simulink model "euler2"  (R2025a)
settings: Solver=VariableStepAuto  StartTime=0.0  StopTime=10.0  RelTol=1e-3
values from neighbouring files (symbols this model uses):
  h = 0.1    [ejemplo_NOlineal_RK4.m]    (also in euler_explicita.m = (tf - t0)/n; euler_explicito.m = (tf - t0)/n; euler_midpoint.m = (tf - t0)/n; examplecrk4.m)
  y0 = 1    [ExampleEuler.m]    (also in ejemplo_NOlineal_RK4.m; examplecrk4.m; exmapleEuler2.m; lineal_RK4.m)
settings Model: Creator=a.diteodoro  LastModifiedBy=a.diteodoro

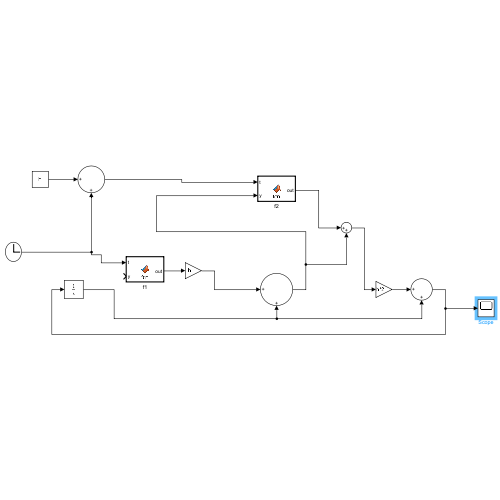
[thumbnail: Simulink's stored preview of the top-level diagram]
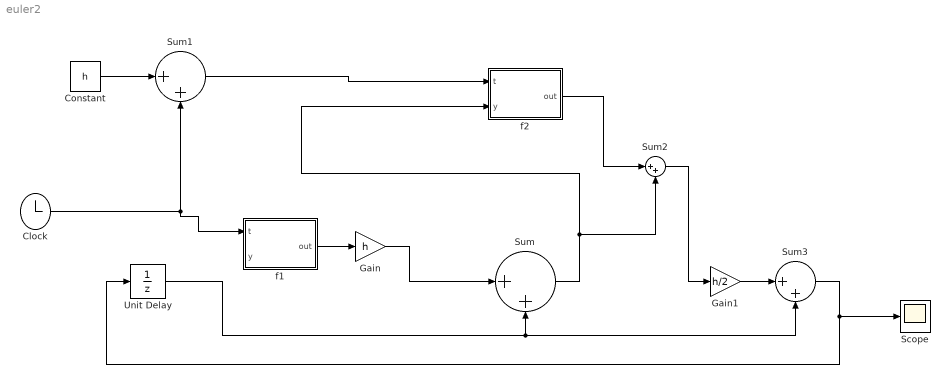
== system euler2 ==
  Clock : Clock
  Constant : Constant  Value=h
  Gain : Gain  Gain=h
  Gain1 : Gain  Gain=h/2
  Scope : Scope
      settings: ActiveDisplayYMinimum=-0.08278445815918023  ActiveDisplayYMaximum=8.8531576900685049
  Sum{,1..3} (4 alike) : Sum  Inputs=|++
  Unit Delay : UnitDelay  InitialCondition=y0  SampleTime=h  HasFrameUpgradeWarning=on
  f1 : MATLAB Function  TreatAsAtomicUnit=on
  f2 : MATLAB Function  TreatAsAtomicUnit=on
  wires:
  Clock/1 -> f1/1(t), Sum1/2
  Unit Delay/1 -> Sum3/2, Sum/2
  Constant/1 -> Sum1/1
  f1/1(out) -> Gain/1
  Sum1/1 -> f2/1(t)
  Gain/1 -> Sum/1
  Sum/1 -> Sum2/2, f2/2(y)
  f2/1(out) -> Sum2/1
  Sum2/1 -> Gain1/1
  Gain1/1 -> Sum3/1
  Sum3/1 -> Unit Delay/1, Scope/1

== matlab function euler2/f1 ==
  data: t input; out output; y input
function out = fcn(t, y)
out = -2*y + t;   % ejemplo
end

== matlab function euler2/f2 ==
  data: t input; out output; y input
function out = fcn(t, y)
out = -2*y + t;   % ejemplo
end
